simulink model "bidirectional converter"  (R2018a)
settings: Solver=ode23t  StartTime=0.0  StopTime=3  RelTol=1e-3
libraries: powerlib x28, simulink x5, re_lib x1
settings Model: Creator=dharun  LastModifiedBy=dharun
settings SolverCC: AlgebraicLoopSolver=LineSearch
settings DataIOCC: ReturnWorkspaceOutputs=on
settings SFSimCC: SimUseLocalCustomCode=on
settings RTWCC: RTWUseLocalCustomCode=on

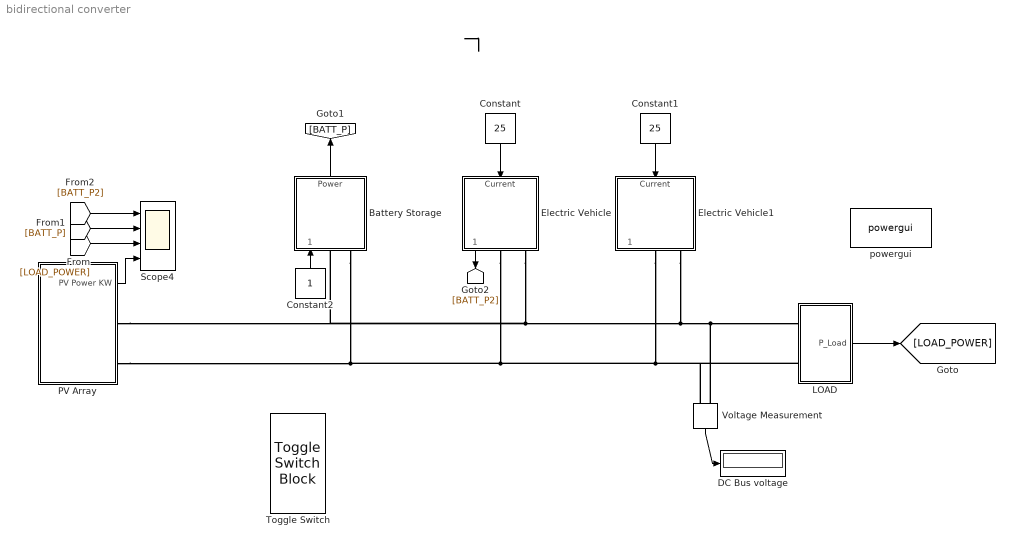
== system bidirectional converter ==
  Battery Storage : Subsystem
  Constant : Constant  Value=25
  Constant1 : Constant  Value=25
  Constant2 : Constant
  DC Bus voltage : Display
  Electric Vehicle : Subsystem
  Electric Vehicle1 : Subsystem
  LOAD : Subsystem
  "PV Array " : Subsystem
  Scope4 : Scope  NumInputPorts=4
  Toggle Switch : ToggleSwitchBlock  WebBlockId=253
      settings: Values={{'Off', 'On'}, [0 1]}
  Voltage Measurement : powerlib/Measurements/Voltage Measurement  PhasorSimulation=off  OutputType=Complex  PSBequivalent=0
      settings: SourceProductName=Simscape Electrical
  powergui : powerlib/powergui  Priority=1  SimulationMode=Discrete  SampleTime=1e-6  frequency=60  Iterations=50  frequencyindice=0  Pbase=100e6  ErrMax=1e-4  UnitsV=kV  UnitsW=MW  buscounter=0  FunctionMessages=off  echomessages=off  EnableUseOfTLC=off  CurrentSourceSwitches=off  DisableSnubberDevices=off  DisableRonSwitches=off  DisableVfSwitches=off  DisplayEquations=off  AutomaticDiscreteSolvers=off  SolverType=Tustin/Backward Euler (TBE)  Interpol=off  ExternalGateDelay=off  methode=off  Ts=100  x0status=blocks  SPID=on  SwTol=0  HookPort=off  NonlinearTolerance=1e-4  nMaxIteration=100  ContinueOnMaxIteration=off  RestoreLinks=warning  ResistiveCurrentMeasurement=off  Frange=[0:2:500]  Ylog=off  Xlog=on  ShowGrid=off  save=off  variable=ZData  structure=0  ZoomFFT=off  StartTime=0.0  cycles=1  DisplayStyle=1  fundamental=60  FreqAxis=off  MaxFrequency=1000  frequencyindicesteady=1  RmsSteady=1  display=off
      settings: SourceProductName=Simscape Electrical
  wires:
  "PV Array "/1(PV Power KW) -> Scope4/4
  [LOAD_POWER] -> Scope4/3
  [BATT_P] -> Scope4/2
  Electric Vehicle/1(" POWER") -> [BATT_P2]
  [BATT_P2] -> Scope4/1
  Battery Storage/1(Power) -> [BATT_P]
  LOAD/1(P_Load) -> [LOAD_POWER]
  Constant/1 -> Electric Vehicle/1(Current)
  Voltage Measurement/1 -> DC Bus voltage/1
  Constant1/1 -> Electric Vehicle1/1(Current)
  Constant2/1 -> Battery Storage/1(Inport)
  connections:
  Electric Vehicle/RConn1 -- Electric Vehicle1/RConn1 -- Voltage Measurement/LConn2 -- LOAD/LConn2 -- "PV Array "/RConn2 -- Battery Storage/LConn2
  Electric Vehicle/RConn2 -- Voltage Measurement/LConn1 -- LOAD/LConn1 -- Electric Vehicle1/RConn2 -- "PV Array "/RConn1 -- Battery Storage/LConn1
  ?

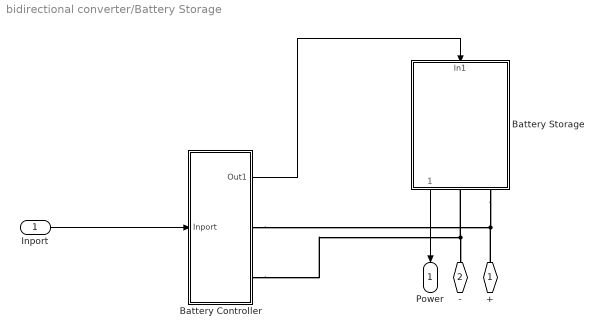
== system bidirectional converter/Battery Storage ==
  Inport : Inport
  Battery Controller : Subsystem
  Battery Storage : Subsystem
  + : PMIOPort  Side=Left
  - : PMIOPort  Port=2  Side=Left
  Power : Outport
  wires:
  Battery Storage/1(BATTERY POWER) -> Power/1
  Battery Controller/1(Out1) -> Battery Storage/1(In1)
  Inport/1 -> Battery Controller/1(Inport)
  connections:
  Battery Controller/RConn1 -- Battery Storage/RConn2 -- +/RConn1
  Battery Controller/RConn2 -- Battery Storage/RConn1 -- -/RConn1

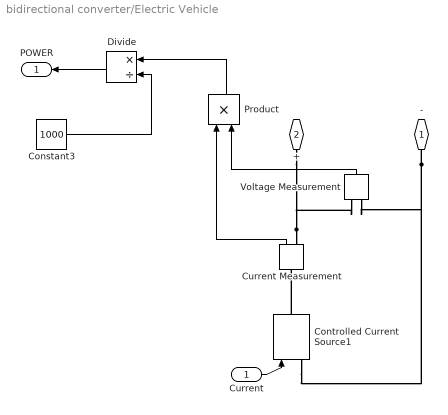
== system bidirectional converter/Electric Vehicle ==
  Current : Inport
  Constant3 : Constant  Value=1000
  Controlled Current Source1 : powerlib/Electrical Sources/Controlled Current Source  Initialize=on  Source_Type=AC  Amplitude=0  Phase=0  Frequency=0  Measurements=None
      settings: SourceProductName=Simscape Electrical
  Current Measurement : powerlib/Measurements/Current Measurement  PhasorSimulation=off  OutputType=Complex  PSBequivalent=0
      settings: SourceProductName=Simscape Electrical
  Divide : Product  Inputs=*/
  Product : Product
  Voltage Measurement : powerlib/Measurements/Voltage Measurement  PhasorSimulation=off  OutputType=Complex  PSBequivalent=0
      settings: SourceProductName=Simscape Electrical
  - : PMIOPort  Side=Right
  + : PMIOPort  Port=2  Side=Right
  " POWER" : Outport
  wires:
  Current/1 -> Controlled Current Source1/1
  Voltage Measurement/1 -> Product/2
  Current Measurement/1 -> Product/1
  Product/1 -> Divide/1
  Constant3/1 -> Divide/2
  Divide/1 -> " POWER"/1
  connections:
  -/RConn1 -- Controlled Current Source1/LConn1 -- Voltage Measurement/LConn2
  Controlled Current Source1/RConn1 -- Current Measurement/LConn1
  Current Measurement/RConn1 -- +/RConn1 -- Voltage Measurement/LConn1

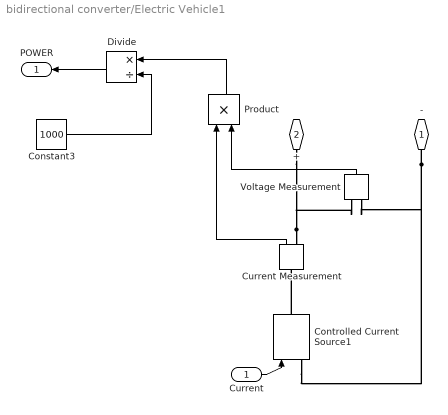
== system bidirectional converter/Electric Vehicle1 ==
  Current : Inport
  Constant3 : Constant  Value=1000
  Controlled Current Source1 : powerlib/Electrical Sources/Controlled Current Source  Initialize=on  Source_Type=AC  Amplitude=0  Phase=0  Frequency=0  Measurements=None
      settings: SourceProductName=Simscape Electrical
  Current Measurement : powerlib/Measurements/Current Measurement  PhasorSimulation=off  OutputType=Complex  PSBequivalent=0
      settings: SourceProductName=Simscape Electrical
  Divide : Product  Inputs=*/
  Product : Product
  Voltage Measurement : powerlib/Measurements/Voltage Measurement  PhasorSimulation=off  OutputType=Complex  PSBequivalent=0
      settings: SourceProductName=Simscape Electrical
  - : PMIOPort  Side=Right
  + : PMIOPort  Port=2  Side=Right
  " POWER" : Outport
  wires:
  Current/1 -> Controlled Current Source1/1
  Voltage Measurement/1 -> Product/2
  Current Measurement/1 -> Product/1
  Product/1 -> Divide/1
  Constant3/1 -> Divide/2
  Divide/1 -> " POWER"/1
  connections:
  -/RConn1 -- Controlled Current Source1/LConn1 -- Voltage Measurement/LConn2
  Controlled Current Source1/RConn1 -- Current Measurement/LConn1
  Current Measurement/RConn1 -- +/RConn1 -- Voltage Measurement/LConn1

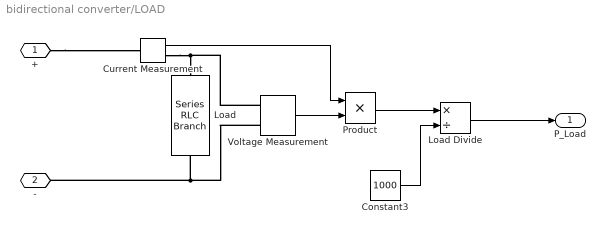
== system bidirectional converter/LOAD ==
  Constant3 : Constant  Value=1000
  Current Measurement : powerlib/Measurements/Current Measurement  PhasorSimulation=off  OutputType=Complex  PSBequivalent=0
      settings: SourceProductName=Simscape Electrical
  Load : powerlib/Elements/Series RLC Branch  LConnTagsString=__new0  RConnTagsString=__new0  BranchType=R  Resistance=1  Inductance=1e-3  SetiL0=off  InitialCurrent=0  Capacitance=1000e-6  Setx0=off  InitialVoltage=0  Measurements=None
      settings: SourceProductName=Simscape Electrical
  Load Divide : Product  Inputs=*/
  Product : Product
  Voltage Measurement : powerlib/Measurements/Voltage Measurement  PhasorSimulation=off  OutputType=Complex  PSBequivalent=0
      settings: SourceProductName=Simscape Electrical
  + : PMIOPort  Side=Left
  - : PMIOPort  Port=2  Side=Left
  P_Load : Outport
  wires:
  Voltage Measurement/1 -> Product/2
  Constant3/1 -> Load Divide/2
  Current Measurement/1 -> Product/1
  Product/1 -> Load Divide/1
  Load Divide/1 -> P_Load/1
  connections:
  +/RConn1 -- Current Measurement/LConn1
  Voltage Measurement/LConn1 -- Load/LConn1 -- Current Measurement/RConn1
  Voltage Measurement/LConn2 -- Load/RConn1 -- -/RConn1

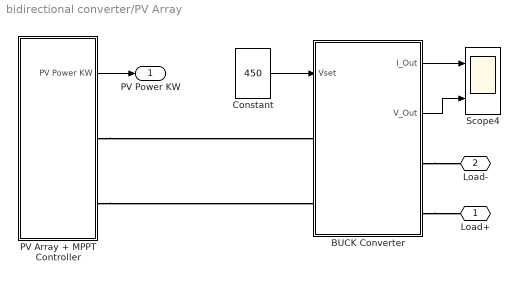
== system bidirectional converter/PV Array  ==
  BUCK Converter : Subsystem
  Constant : Constant  Value=450
  PV Array + MPPT Controller : Subsystem
  Scope4 : Scope  NumInputPorts=2
  Load+ : PMIOPort  Side=Right
  Load- : PMIOPort  Port=2  Side=Right
  PV Power KW : Outport
  wires:
  BUCK Converter/1(I_Out) -> Scope4/1
  BUCK Converter/2(V_Out) -> Scope4/2
  Constant/1 -> BUCK Converter/1(Vset)
  PV Array + MPPT Controller/1("PV Power KW ") -> PV Power KW/1
  connections:
  BUCK Converter/RConn1 -- Load-/RConn1
  BUCK Converter/RConn2 -- Load+/RConn1
  PV Array + MPPT Controller/RConn1 -- BUCK Converter/LConn1
  PV Array + MPPT Controller/RConn2 -- BUCK Converter/LConn2

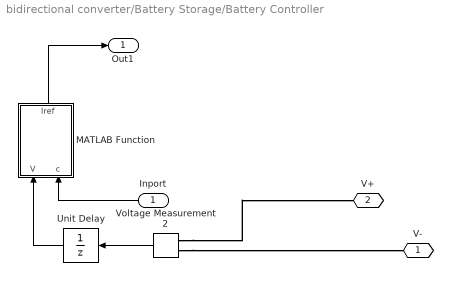
== system bidirectional converter/Battery Storage/Battery Controller ==
  Inport : Inport
  MATLAB Function : MATLAB Function  TreatAsAtomicUnit=on
  Unit Delay : UnitDelay  SampleTime=0.00001  HasFrameUpgradeWarning=on
  Voltage Measurement2 : powerlib/Measurements/Voltage Measurement  PhasorSimulation=off  OutputType=Complex  PSBequivalent=0
      settings: SourceProductName=Simscape Electrical
  V- : PMIOPort  Side=Right
  V+ : PMIOPort  Port=2  Side=Right
  Out1 : Outport
  wires:
  Unit Delay/1 -> MATLAB Function/1(V)
  Voltage Measurement2/1 -> Unit Delay/1
  MATLAB Function/1(Iref) -> Out1/1
  Inport/1 -> MATLAB Function/2(c)
  connections:
  Voltage Measurement2/LConn1 -- V-/RConn1
  Voltage Measurement2/LConn2 -- V+/RConn1

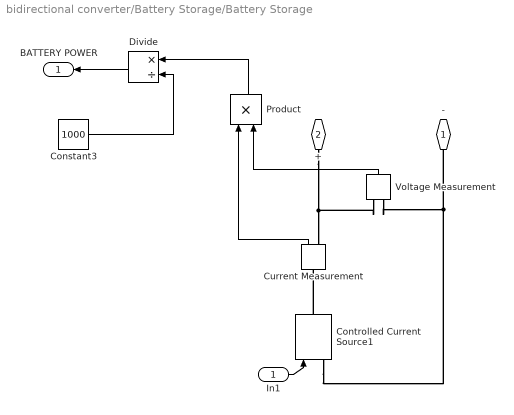
== system bidirectional converter/Battery Storage/Battery Storage ==
  In1 : Inport
  Constant3 : Constant  Value=1000
  Controlled Current Source1 : powerlib/Electrical Sources/Controlled Current Source  Initialize=on  Source_Type=AC  Amplitude=0  Phase=0  Frequency=0  Measurements=None
      settings: SourceProductName=Simscape Electrical
  Current Measurement : powerlib/Measurements/Current Measurement  PhasorSimulation=off  OutputType=Complex  PSBequivalent=0
      settings: SourceProductName=Simscape Electrical
  Divide : Product  Inputs=*/
  Product : Product
  Voltage Measurement : powerlib/Measurements/Voltage Measurement  PhasorSimulation=off  OutputType=Complex  PSBequivalent=0
      settings: SourceProductName=Simscape Electrical
  - : PMIOPort  Side=Right
  + : PMIOPort  Port=2  Side=Right
  BATTERY POWER : Outport
  wires:
  In1/1 -> Controlled Current Source1/1
  Voltage Measurement/1 -> Product/2
  Current Measurement/1 -> Product/1
  Product/1 -> Divide/1
  Constant3/1 -> Divide/2
  Divide/1 -> BATTERY POWER/1
  connections:
  Controlled Current Source1/LConn1 -- Voltage Measurement/LConn2 -- -/RConn1
  Controlled Current Source1/RConn1 -- Current Measurement/LConn1
  +/RConn1 -- Voltage Measurement/LConn1 -- Current Measurement/RConn1

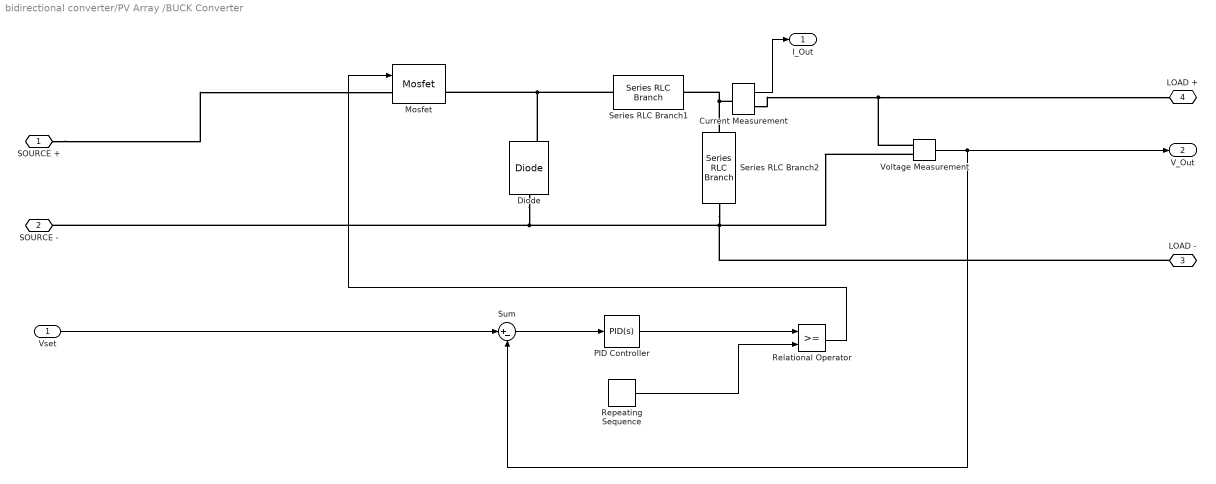
== system bidirectional converter/PV Array /BUCK Converter ==
  Vset : Inport
  Current Measurement : powerlib/Measurements/Current Measurement  PhasorSimulation=off  OutputType=Complex  PSBequivalent=0
      settings: SourceProductName=Simscape Electrical
  Diode : powerlib/Power Electronics/Diode  Ron=0.000001  Lon=0  Vf=0.007  IC=0  UseSnubber=0  Rs=500  Cs=250e-9  Measurements=on
      settings: SourceProductName=Simscape Electrical
  Mosfet : powerlib/Power Electronics/Mosfet  Ron=0.1  Lon=0  Rd=0.0001  Vfd=0  IC=0  Rs=1e5  Cs=inf  Measurements=on
      settings: SourceProductName=Simscape Electrical
  PID Controller : simulink/Continuous/PID Controller  Controller=PID  Form=Parallel  TimeDomain=Continuous-time  SampleTime=-1  IntegratorMethod=Forward Euler  FilterMethod=Forward Euler  ControllerParametersSource=internal  P=50  I=0.5  D=0  UseFilter=on  N=100  TunerSelectOption=Transfer Function Based (PID Tuner App)  InitialConditionSource=internal  InitialConditionForIntegrator=0  InitialConditionForFilter=0  DifferentiatorICPrevScaledInput=0  ExternalReset=none  TrackingMode=off  Kt=1  LimitOutput=on  UpperSaturationLimit=1  LowerSaturationLimit=0  LinearizeAsGain=on  AntiWindupMode=none  Kb=1  POutMin=[]  POutMax=[]  IOutMin=[]  IOutMax=[]  DOutMin=[]  DOutMax=[]  NOutMin=[]  NOutMax=[]  SumOutMin=[]  SumOutMax=[]  SaturationOutMin=[]  SaturationOutMax=[]  PParamMin=[]  PParamMax=[]  IParamMin=[]  IParamMax=[]  DParamMin=[]  DParamMax=[]  NParamMin=[]  NParamMax=[]  KbParamMin=[]  KbParamMax=[]  KtParamMin=[]  KtParamMax=[]  KbOutMin=[]  KbOutMax=[]  KtOutMin=[]  KtOutMax=[]  IntegratorOutMin=[]  IntegratorOutMax=[]  FilterOutMin=[]  FilterOutMax=[]  SumI1OutMin=[]  SumI1OutMax=[]  SumI2OutMin=[]  SumI2OutMax=[]  SumI3OutMin=[]  SumI3OutMax=[]  SumDOutMin=[]  SumDOutMax=[]  DifferentiatorOutMin=[]  DifferentiatorOutMax=[]  FilterDiffOutCoefMin=[]  FilterDiffOutCoefMax=[]  ReciprocalOutMin=[]  ReciprocalOutMax=[]  SumDenOutMin=[]  SumDenOutMax=[]  SumNumOutMin=[]  SumNumOutMax=[]  DivideOutMin=[]  DivideOutMax=[]  IntegratorContinuousStateAttributes=''  IntegratorStateMustResolveToSignalObject=off  IntegratorRTWStateStorageClass=Auto  FilterContinuousStateAttributes=''  FilterStateMustResolveToSignalObject=off  FilterRTWStateStorageClass=Auto
  Relational Operator : RelationalOperator  OutDataTypeStr=boolean  RndMeth=Simplest
  Repeating Sequence : simulink/Sources/Repeating Sequence  rep_seq_t=[0 0.00004]  rep_seq_y=[0 1]
  Series RLC Branch1 : powerlib/Elements/Series RLC Branch  LConnTagsString=__new0  RConnTagsString=__new0  BranchType=L  Resistance=1  Inductance=145e-6  SetiL0=off  InitialCurrent=0  Capacitance=1e-6  Setx0=off  InitialVoltage=0  Measurements=None
      settings: SourceProductName=Simscape Electrical
  Series RLC Branch2 : powerlib/Elements/Series RLC Branch  LConnTagsString=__new0  RConnTagsString=__new0  BranchType=C  Resistance=1  Inductance=1e-3  SetiL0=off  InitialCurrent=0  Capacitance=2000e-6  Setx0=off  InitialVoltage=0  Measurements=None
      settings: SourceProductName=Simscape Electrical
  Sum : Sum  Inputs=|+-
  Voltage Measurement : powerlib/Measurements/Voltage Measurement  PhasorSimulation=off  OutputType=Complex  PSBequivalent=0
      settings: SourceProductName=Simscape Electrical
  SOURCE + : PMIOPort  Side=Left
  SOURCE - : PMIOPort  Port=2  Side=Left
  LOAD - : PMIOPort  Port=3  Side=Right
  LOAD + : PMIOPort  Port=4  Side=Right
  I_Out : Outport
  V_Out : Outport  Port=2
  wires:
  Vset/1 -> Sum/1
  Sum/1 -> PID Controller/1
  Repeating Sequence/1 -> Relational Operator/2
  Current Measurement/1 -> I_Out/1
  Voltage Measurement/1 -> V_Out/1, Sum/2
  PID Controller/1 -> Relational Operator/1
  Relational Operator/1 -> Mosfet/1
  connections:
  SOURCE +/RConn1 -- Mosfet/LConn1
  Voltage Measurement/LConn1 -- Current Measurement/RConn1 -- LOAD +/RConn1
  Current Measurement/LConn1 -- Series RLC Branch1/RConn1 -- Series RLC Branch2/LConn1
  Diode/LConn1 -- LOAD -/RConn1 -- Voltage Measurement/LConn2 -- Series RLC Branch2/RConn1 -- SOURCE -/RConn1
  Series RLC Branch1/LConn1 -- Diode/RConn1 -- Mosfet/RConn1

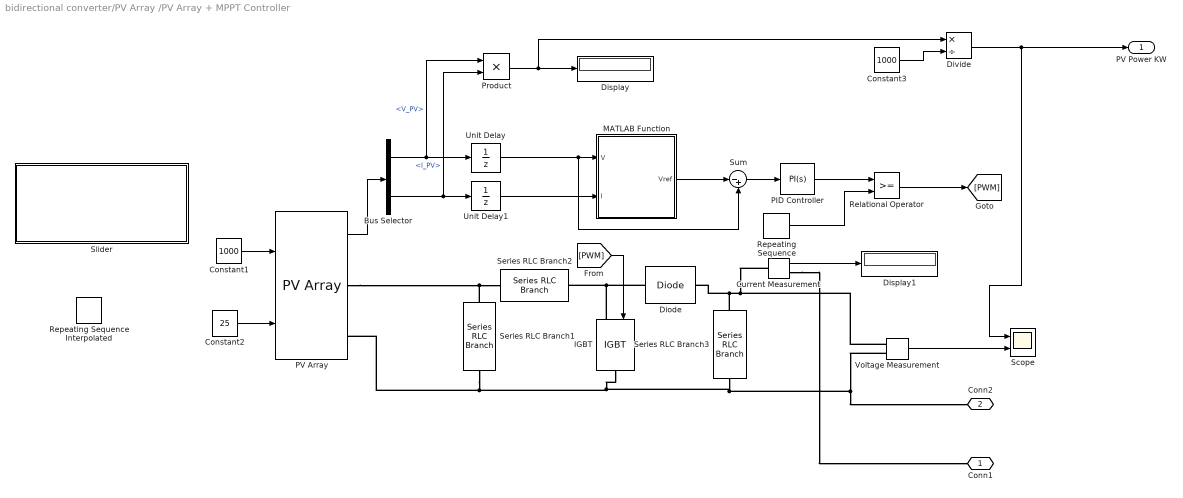
== system bidirectional converter/PV Array /PV Array + MPPT Controller ==
  Bus Selector : BusSelector  OutputSignals=V_PV,I_PV
  Constant1 : Constant  Value=1000
  Constant2 : Constant  Value=25
  Constant3 : Constant  Value=1000
  Current Measurement : powerlib/Measurements/Current Measurement  PhasorSimulation=off  OutputType=Complex  PSBequivalent=0
      settings: SourceProductName=Simscape Electrical
  Diode : powerlib/Power Electronics/Diode  Ron=0.001  Lon=0  Vf=0.8  IC=0  UseSnubber=0  Rs=500  Cs=250e-9  Measurements=off
      settings: SourceProductName=Simscape Electrical
  Display : Display
  Display1 : Display
  Divide : Product  Inputs=*/
  IGBT : powerlib/Power Electronics/IGBT  Ron=0.001  Lon=0  Vf=1  Tf=1e-6  Tt=2e-6  IC=0  Rs=1e5  Cs=inf  Measurements=off
      settings: SourceProductName=Simscape Electrical
  MATLAB Function : MATLAB Function  TreatAsAtomicUnit=on
  PID Controller : simulink/Continuous/PID Controller  Controller=PI  Form=Parallel  TimeDomain=Continuous-time  SampleTime=-1  IntegratorMethod=Forward Euler  FilterMethod=Forward Euler  ControllerParametersSource=internal  P=0.0005  I=0.01  D=0  UseFilter=on  N=100  TunerSelectOption=Transfer Function Based (PID Tuner App)  InitialConditionSource=internal  InitialConditionForIntegrator=0  InitialConditionForFilter=0  DifferentiatorICPrevScaledInput=0  ExternalReset=none  TrackingMode=off  Kt=1  LimitOutput=on  UpperSaturationLimit=0.95  LowerSaturationLimit=0  LinearizeAsGain=on  AntiWindupMode=none  Kb=1  POutMin=[]  POutMax=[]  IOutMin=[]  IOutMax=[]  DOutMin=[]  DOutMax=[]  NOutMin=[]  NOutMax=[]  SumOutMin=[]  SumOutMax=[]  SaturationOutMin=[]  SaturationOutMax=[]  PParamMin=[]  PParamMax=[]  IParamMin=[]  IParamMax=[]  DParamMin=[]  DParamMax=[]  NParamMin=[]  NParamMax=[]  KbParamMin=[]  KbParamMax=[]  KtParamMin=[]  KtParamMax=[]  KbOutMin=[]  KbOutMax=[]  KtOutMin=[]  KtOutMax=[]  IntegratorOutMin=[]  IntegratorOutMax=[]  FilterOutMin=[]  FilterOutMax=[]  SumI1OutMin=[]  SumI1OutMax=[]  SumI2OutMin=[]  SumI2OutMax=[]  SumI3OutMin=[]  SumI3OutMax=[]  SumDOutMin=[]  SumDOutMax=[]  DifferentiatorOutMin=[]  DifferentiatorOutMax=[]  FilterDiffOutCoefMin=[]  FilterDiffOutCoefMax=[]  ReciprocalOutMin=[]  ReciprocalOutMax=[]  SumDenOutMin=[]  SumDenOutMax=[]  SumNumOutMin=[]  SumNumOutMax=[]  DivideOutMin=[]  DivideOutMax=[]  IntegratorContinuousStateAttributes=''  IntegratorStateMustResolveToSignalObject=off  IntegratorRTWStateStorageClass=Auto  FilterContinuousStateAttributes=''  FilterStateMustResolveToSignalObject=off  FilterRTWStateStorageClass=Auto
  PV Array : re_lib/Solar/PV Array  Npar=47  Nser=10  PlotType=array @ 25 deg.C & specified irradiances  S_vec="[ 1000  500  100 ]"  Temp_C_vec="[ 45 25  ]"  ModuleName=1Soltech 1STH-215-P  PlotWhenSelected=off  Pm=213.15  Ncell=60  Voc=36.3  Isc=7.84  Vm=29  Im=7.35  beta_Voc_pc=-0.36099  alpha_Isc_pc=0.102  beta_Voc=-0.13104  alpha_Isc=0.007997  IL=7.8649  I0=2.9259e-10  nI=0.98117  Rsh=313.3991  Rs=0.39383  BAL=off  Tc=1e-6  Tfilter=5e-5
      settings: SourceProductName=Simscape Electrical
  Product : Product
  Relational Operator : RelationalOperator  OutDataTypeStr=boolean  RndMeth=Simplest
  Repeating Sequence : simulink/Sources/Repeating Sequence  rep_seq_t=[0 0.0002]  rep_seq_y=[0 1]
  Repeating Sequence Interpolated : simulink/Sources/Repeating Sequence Interpolated  OutValues="[1000 700  900 1000].'"  TimeValues=[0.5 1 1.5 2.5 ].'  LookUpMeth=Interpolation-Use End Values  tsamp=0.01  OutMin=[]  OutMax=[]  OutDataTypeStr=double  OutputDataTypeScalingMode=double  OutDataType=fixdt(0,8)  OutScaling=2^-10
  Scope : Scope  NumInputPorts=2
  Series RLC Branch1 : powerlib/Elements/Series RLC Branch  LConnTagsString=__new0  RConnTagsString=__new0  BranchType=RC  Resistance=0.0001  Inductance=1e-3  SetiL0=off  InitialCurrent=0  Capacitance=1000e-6  Setx0=off  InitialVoltage=0  Measurements=None
      settings: SourceProductName=Simscape Electrical
  Series RLC Branch2 : powerlib/Elements/Series RLC Branch  LConnTagsString=__new0  RConnTagsString=__new0  BranchType=L  Resistance=0.0001  Inductance=1.45e-3  SetiL0=off  InitialCurrent=0  Capacitance=1000e-6  Setx0=off  InitialVoltage=0  Measurements=None
      settings: SourceProductName=Simscape Electrical
  Series RLC Branch3 : powerlib/Elements/Series RLC Branch  LConnTagsString=__new0  RConnTagsString=__new0  BranchType=C  Resistance=0.0001  Inductance=1e-3  SetiL0=off  InitialCurrent=0  Capacitance=3227e-6  Setx0=off  InitialVoltage=0  Measurements=None
      settings: SourceProductName=Simscape Electrical
  Slider : Subsystem  DialogController=hmiCreateDDGDialog  IsWebBlock=on  mask(MWDashboardBlock){webBlockId=24c7ad11-1b97-4736-b433-52eee7e6992b, webBlockType=slider, ShowInLibBrowser=on, ShowInitialText=on, HMISrcModelName=Final_Project_Stage4}
      mask prompts: webBlockId "WebBlock Id"; webBlockType "WebBlock Type"; HMISrcModelName "Source Model"
      mask help: Set value to tune parameters or variables.
      mask Help: helpview([docroot '/mapfiles/simulink.map'], 'hmi_slider')
      mask Display:
      | if strcmp(get_param(bdroot(gcb),'BlockDiagramType'),'library')
      |  image([(matlabroot) '/toolbox/simulink/hmi/icons/Slider.png'])
      | end
  Sum : Sum  Inputs=|-+
  Unit Delay : UnitDelay  SampleTime=1e-4  HasFrameUpgradeWarning=on
  Unit Delay1 : UnitDelay  SampleTime=1e-4  HasFrameUpgradeWarning=on
  Voltage Measurement : powerlib/Measurements/Voltage Measurement  PhasorSimulation=off  OutputType=Complex  PSBequivalent=0
      settings: SourceProductName=Simscape Electrical
  Conn1 : PMIOPort  Side=Right
  Conn2 : PMIOPort  Port=2  Side=Right
  "PV Power KW " : Outport
  wires:
  Repeating Sequence/1 -> Relational Operator/2
  Relational Operator/1 -> [PWM]
  Constant3/1 -> Divide/2
  Constant1/1 -> PV Array/1
  Unit Delay/1 -> Sum/2, MATLAB Function/1(V)
  Unit Delay1/1 -> MATLAB Function/2(I)
  PID Controller/1 -> Relational Operator/1
  Constant2/1 -> PV Array/2
  PV Array/1 -> Bus Selector/1
  Divide/1 -> Scope/1, "PV Power KW "/1
  Voltage Measurement/1 -> Scope/2
  Product/1 -> Divide/1, Display/1
  Bus Selector/1 -> Product/1, Unit Delay/1  "<V_PV>"
  Current Measurement/1 -> Display1/1
  [PWM] -> IGBT/1
  Sum/1 -> PID Controller/1
  Bus Selector/2 -> Product/2, Unit Delay1/1  "<I_PV>"
  MATLAB Function/1(Vref) -> Sum/1
  connections:
  Current Measurement/RConn1 -- Conn1/RConn1
  PV Array/RConn1 -- Series RLC Branch1/LConn1 -- Series RLC Branch2/RConn1
  Series RLC Branch1/RConn1 -- Voltage Measurement/LConn2 -- Conn2/RConn1 -- Series RLC Branch3/RConn1 -- IGBT/RConn1 -- PV Array/RConn2
  Series RLC Branch3/LConn1 -- Current Measurement/LConn1 -- Voltage Measurement/LConn1 -- Diode/RConn1
  IGBT/LConn1 -- Diode/LConn1 -- Series RLC Branch2/LConn1

== system bidirectional converter/PV Array /PV Array + MPPT Controller/Slider ==

== matlab function bidirectional converter/Battery Storage/Battery Controller/MATLAB Function ==
  data: V input; Iref output; c input
function Iref = RefGen(V,c)

persistent Iold ;

if isempty(Iold)
    Iold = 0;
end

if c==1
    
if V<=450 
    Iref=Iold+0.01;
elseif V>450
    Iref=Iold-0.01;
else
    Iref=Iold;
end

else
    Iref=0;

end
Iold = Iref;

== matlab function bidirectional converter/PV Array /PV Array + MPPT Controller/MATLAB Function ==
  data: V input; Vref output; I input
function Vref = RefGen(V, I)

Vrefmax =363;
Vrefmin=0;
Vrefinit=300;
deltaVref=1;

persistent Vold Pold Vrefold;

dataType = 'double';

if isempty(Vold)
    Vold = 0;
    Pold = 0;
    Vrefold=Vrefinit;
end

P = V*I;
dV = V-Vold;
dP = P-Pold;

if dP ~= 0
    if dP<0
        if dV<0
            Vref=Vrefold+deltaVref;
        else 
            Vref= Vrefold-deltaVref;
        end
    else
        if dV<0
            Vref=Vrefold-deltaVref;
        else
            Vref=Vrefold+deltaVref;
        end
    end
else  Vref = Vrefold;
end

if Vref >= Vrefmax || Vref<=Vrefmin || V>= 600
    Vref = Vrefold;
end

Vrefold = Vref;
Vold = V;
Pold = P;
